simulink model "almost_round"  (R2017b)
settings: Solver=ode45  StartTime=0.0  StopTime=time_end  RelTol=1e-3  EnableMultiTasking=on
values from neighbouring files (symbols this model uses):
  alpha_initial = 0    [run.m]
  g = 9.8    [run.m]
  gamma = (k)/(2*m*r)    (= 6.57462195924)    [run.m]
  k = 0.8    [run.m]
  m = 0.078    [run.m]
  sample_time = 0.1    [run.m]
  W_initial = 0    [run.m]
  x_initial = 0.5    [run.m]
  z_initial = 0.5    [run.m]
undefined symbols (not defined in the file or in its folder): magnitude
settings Model: Creator=Subject 1482  LastModifiedBy=Subject 1482
settings DataIOCC: LimitDataPoints=on  SaveFormat=Array
settings OptimizationCC: LifeSpan=inf
settings DebuggingCC: SFUnexpectedBacktrackingDiag=warning  SFNoUnconditionalDefaultTransitionDiag=warning  SFExecutionAtInitializationDiag=none
settings HardwareCC: ProdBitPerPointer=32  ProdBitPerSizeT=32  ProdBitPerPtrDiffT=32  ProdLargestAtomicFloat=None  ProdIntDivRoundTo=Undefined  ProdEndianess=Unspecified  ProdWordSize=32  ProdHWDeviceType=32-bit Generic
settings ModelReferenceCC: PropagateSignalLabelsOutOfModel=off
settings CodeAppCC: StateflowObjectComments=on
settings GRTTargetCC: TargetLangStandard=C89/C90 (ANSI)  GeneratePreprocessorConditionals=Disable all
settings ConfigComp: CovMetricSettings=dw  CovHtmlReporting=on  CovSaveCumulativeToWorkspaceVar=on  CovSaveSingleToWorkspaceVar=on  CovExternalEMLEnable=off

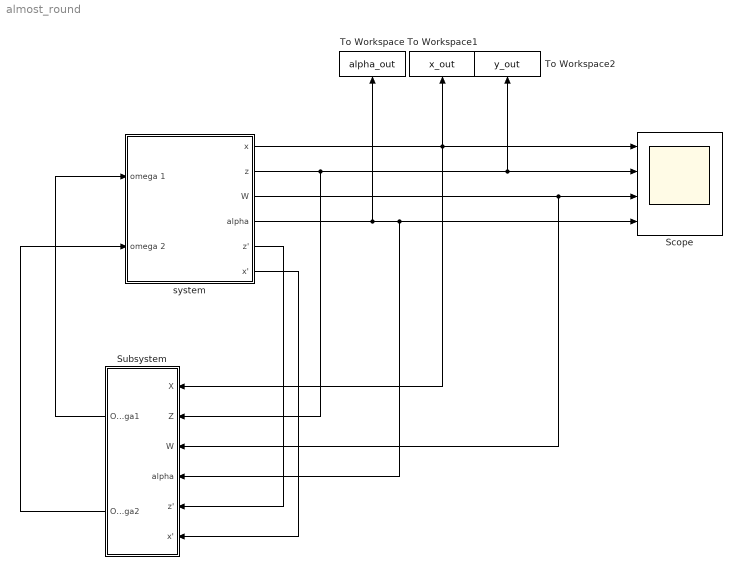
== system almost_round ==
  Scope : Scope  NumInputPorts=4
  Subsystem : Subsystem
  To Workspace : ToWorkspace  VariableName=alpha_out  SaveFormat=Timeseries  SampleTime=sample_time
  To Workspace1 : ToWorkspace  VariableName=x_out  SaveFormat=Timeseries  SampleTime=sample_time
  To Workspace2 : ToWorkspace  VariableName=y_out  SaveFormat=Timeseries  SampleTime=sample_time
  system : Subsystem
  wires:
  system/4(alpha) -> To Workspace/1, Subsystem/4(alpha), Scope/4
  system/2(z) -> To Workspace2/1, Scope/2, Subsystem/2(Z)
  system/1(x) -> Subsystem/1(X), Scope/1, To Workspace1/1
  system/3(W) -> Scope/3, Subsystem/3(W)
  system/5(z') -> Subsystem/5(z')
  system/6(x') -> Subsystem/6(x')
  Subsystem/1(Omega1) -> system/1(omega 1)
  Subsystem/2(Omega2) -> system/2(omega 2)

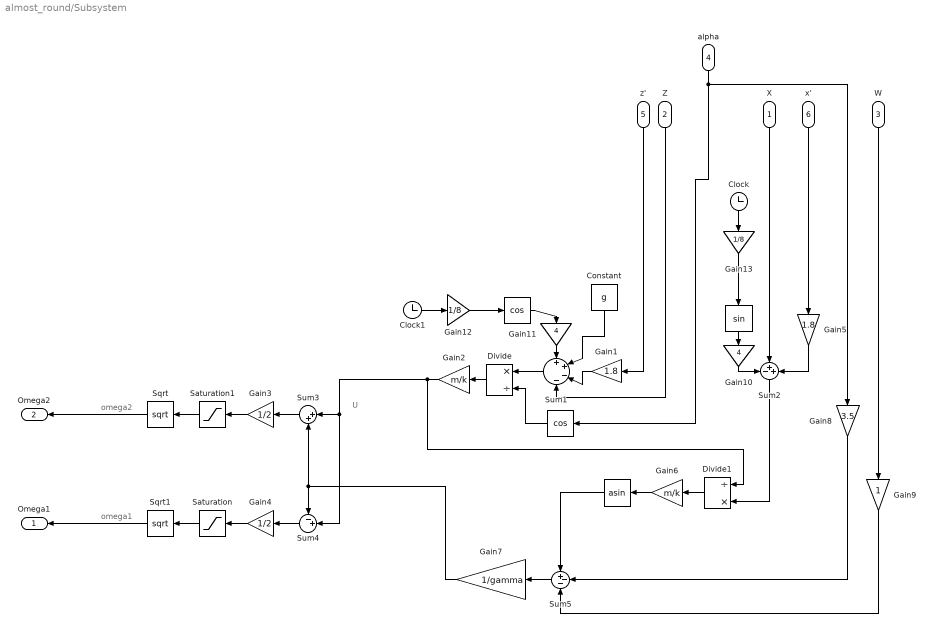
== system almost_round/Subsystem ==
  note: omega1
  note: omega2
  note: U
  X : Inport
  Z : Inport  Port=2
  W : Inport  Port=3
  alpha : Inport  Port=4
  z' : Inport  Port=5
  x' : Inport  Port=6
  " " : Trigonometry  Operator=cos
  "   " : Trigonometry  Operator=asin
  "    " : Trigonometry
  "        " : Trigonometry  Operator=cos
  Clock : Clock
  Clock1 : Clock
  Constant : Constant  Value=g
  Divide : Product  Inputs=*/
  Divide1 : Product  Inputs=/*
  Gain1 : Gain  Gain=1.8
  Gain10 : Gain  Gain=4
  Gain11 : Gain  Gain=4
  Gain12 : Gain  Gain=1/8
  Gain13 : Gain  Gain=1/8
  Gain2 : Gain  Gain=m/k
  Gain3 : Gain  Gain=1/2
  Gain4 : Gain  Gain=1/2
  Gain5 : Gain  Gain=1.8
  Gain6 : Gain  Gain=m/k
  Gain7 : Gain  Gain=1/gamma
  Gain8 : Gain  Gain=3.5
  Gain9 : Gain
  Saturation : Saturate  UpperLimit=1000  LowerLimit=0.0001
  Saturation1 : Saturate  UpperLimit=1000  LowerLimit=0.0001
  Sqrt : Sqrt  SaturateOnIntegerOverflow=on
  Sqrt1 : Sqrt  SaturateOnIntegerOverflow=on
  Sum1 : Sum  Inputs=++--
  Sum2 : Sum  Inputs=-++
  Sum3 : Sum  Inputs=|++
  Sum4 : Sum  Inputs=-+|
  Sum5 : Sum  Inputs=+--
  Omega1 : Outport
  Omega2 : Outport  Port=2
  wires:
  Sum3/1 -> Gain3/1
  Saturation1/1 -> Sqrt/1
  Sqrt1/1 -> Omega1/1
  Sum4/1 -> Gain4/1
  Gain4/1 -> Saturation/1
  Gain3/1 -> Saturation1/1
  Sqrt/1 -> Omega2/1
  Saturation/1 -> Sqrt1/1
  Gain2/1 -> Divide1/1, Sum3/1, Sum4/2
  Constant/1 -> Sum1/2
  z'/1 -> Gain1/1
  Sum1/1 -> Divide/1
  " "/1 -> Divide/2
  Divide/1 -> Gain2/1
  Gain1/1 -> Sum1/3
  Sum2/1 -> Divide1/2
  Divide1/1 -> Gain6/1
  x'/1 -> Gain5/1
  Gain5/1 -> Sum2/3
  Gain7/1 -> Sum3/2, Sum4/1
  Sum5/1 -> Gain7/1
  Gain8/1 -> Sum5/2
  Gain6/1 -> "   "/1
  "   "/1 -> Sum5/1
  Clock/1 -> Gain13/1
  Clock1/1 -> Gain12/1
  Gain9/1 -> Sum5/3
  "    "/1 -> Gain10/1
  Gain10/1 -> Sum2/1
  Gain11/1 -> Sum1/1
  "        "/1 -> Gain11/1
  Gain12/1 -> "        "/1
  Gain13/1 -> "    "/1
  alpha/1 -> " "/1, Gain8/1
  W/1 -> Gain9/1
  X/1 -> Sum2/2
  Z/1 -> Sum1/4

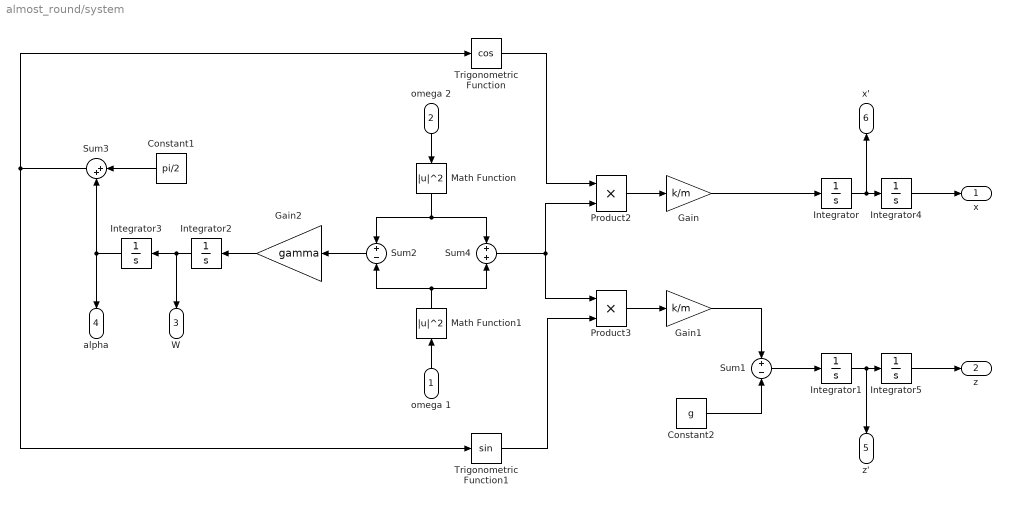
== system almost_round/system ==
  omega 1 : Inport
  omega 2 : Inport  Port=2
  Constant1 : Constant  Value=pi/2
  Constant2 : Constant  Value=g
  Gain : Gain  Gain=k/m
  Gain1 : Gain  Gain=k/m
  Gain2 : Gain  Gain=gamma
  Integrator : Integrator
  Integrator1 : Integrator
  Integrator2 : Integrator  InitialCondition=W_initial
  Integrator3 : Integrator  InitialCondition=alpha_initial
  Integrator4 : Integrator  InitialCondition=x_initial
  Integrator5 : Integrator  InitialCondition=z_initial
  Math Function : Math  Operator=magnitude^2  SaturateOnIntegerOverflow=on
  Math Function1 : Math  Operator=magnitude^2  SaturateOnIntegerOverflow=on
  Product2 : Product
  Product3 : Product
  Sum1 : Sum  Inputs=+-
  Sum2 : Sum  Inputs=+-
  Sum3 : Sum  Inputs=|++
  Sum4 : Sum
  Trigonometric Function : Trigonometry  Operator=cos
  Trigonometric Function1 : Trigonometry
  x : Outport
  z : Outport  Port=2
  W : Outport  Port=3
  alpha : Outport  Port=4
  z' : Outport  Port=5
  x' : Outport  Port=6
  wires:
  Constant2/1 -> Sum1/2
  Gain1/1 -> Sum1/1
  Sum1/1 -> Integrator1/1
  Product3/1 -> Gain1/1
  Trigonometric Function/1 -> Product2/1
  Gain2/1 -> Integrator2/1
  Integrator3/1 -> Sum3/2, alpha/1
  Trigonometric Function1/1 -> Product3/2
  Product2/1 -> Gain/1
  Gain/1 -> Integrator/1
  Integrator2/1 -> W/1, Integrator3/1
  Constant1/1 -> Sum3/1
  Sum3/1 -> Trigonometric Function1/1, Trigonometric Function/1
  Integrator1/1 -> z'/1, Integrator5/1
  Integrator5/1 -> z/1
  Integrator/1 -> x'/1, Integrator4/1
  Integrator4/1 -> x/1
  Sum2/1 -> Gain2/1
  Sum4/1 -> Product3/1, Product2/2
  omega 2/1 -> Math Function/1
  Math Function/1 -> Sum2/1, Sum4/1
  Math Function1/1 -> Sum4/2, Sum2/2
  omega 1/1 -> Math Function1/1
